simulink model "darko_control_lineaire_lqi"  (R2020b)
settings: Solver=VariableStepAuto  StartTime=0.0  StopTime=30  RelTol=1e-3
values from neighbouring files (symbols this model uses):
  drone = generateDarko()    [main_linearisation_rot.m]
  initial_state = [p_initial; v_initial; q_initial; omega_initial]    [main_linearisation_rot.m]
  K_complet_i = [Ki(:,1:6), zeros(4,1), Ki(:,7:15)]    [main_linearisation_rot.m]
  S_complet_i = [Si(1:6,1:6), zeros(6,1), Si(1:6,7:15); zeros(1,16); Si(7:15,1:6), zeros(9,1), Si(7:15,7:15)]    [main_linearisation_rot.m]
  u_eq = drone.G*drone.MASS/(2*drone.Fb(1,1)) * [1;1;0;0]    [main_linearisation_rot.m]
  x_eq = [[0; 0; 0]; [0; 0; 0]; [1/sqrt(2); 0; -1/sqrt(2);0]; [0; 0; 0]]    [main_linearisation_rot.m]
libraries: simulink_extras x5, aerolibanim x1, sharedtransform x1
settings Model: Creator=florian  LastModifiedBy=florian

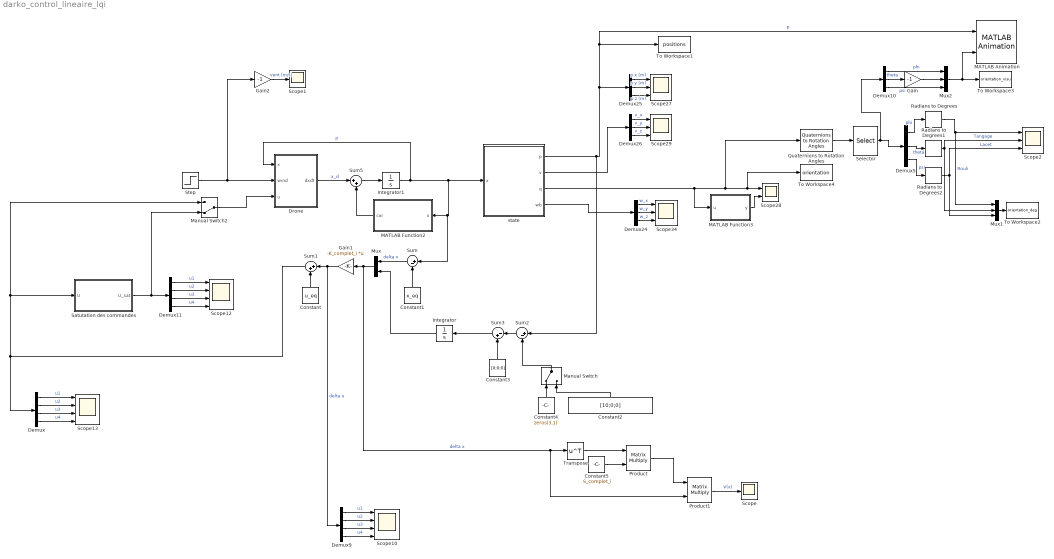
== system darko_control_lineaire_lqi ==
  Constant : Constant  Value=u_eq
  Constant1 : Constant  Value=x_eq
  Constant2 : Constant  Value=[10;0;0]
  Constant3 : Constant  Value=[0;0;0]
  Constant4 : Constant  Value=zeros(3,1)
  Constant5 : Constant  Value=S_complet_i
  Demux : Demux
  Demux{5,10,24..26} (5 alike) : Demux  Outputs=3
  Demux11 : Demux
  Demux9 : Demux
  Drone : MATLAB Function  TreatAsAtomicUnit=on
  Gain : Gain  Gain=-1
  Gain1 : Gain  Gain=-K_complet_i  Multiplication=Matrix(K*u) (u vector)
  Gain2 : Gain  Gain=-1
  Integrator : Integrator  InitialCondition=[0;0;0]
  Integrator1 : Integrator  InitialCondition=initial_state
  MATLAB Animation : aerolibanim/MATLAB Animation  Tag=Matlab Animation 6 DOF  Vehicles=1  Geometries='astredwedge.mat'  BoundingBoxCoordinates=[-50,50,-50,50,-50,50]  CameraOffset=[0,-50,0]  CameraViewAngle=10  SampleTime=0.08  FigurePosition=[635,-23,492,413]
      settings: SourceProductBaseCode=AE
  MATLAB Function2 : MATLAB Function  TreatAsAtomicUnit=on
  MATLAB Function3 : MATLAB Function  TreatAsAtomicUnit=on
  Manual Switch : ManualSwitch
  Manual Switch2 : ManualSwitch  CurrentSetting=0
  Mux : Mux  Inputs=2
  Mux1 : Mux  Inputs=3
  Mux2 : Mux  Inputs=3
  Product : Product  Multiplication=Matrix(*)
  Product1 : Product  Multiplication=Matrix(*)
  Quaternions to Rotation Angles : sharedtransform/Quaternions to Rotation Angles  rotationOrder=ZXY  aMode=aMode
      settings: SourceProductBaseCode=AE,PW,MT,UV,VE,VP
  Radians to Degrees : simulink_extras/Transformations/Radians to Degrees
  Radians to Degrees1 : simulink_extras/Transformations/Radians to Degrees
  Radians to Degrees2 : simulink_extras/Transformations/Radians to Degrees
  Satutation des commandes : Subsystem
  Scope : Scope
  Scope1 : Scope
  Scope10 : Scope  NumInputPorts=4
  Scope12 : Scope  NumInputPorts=4
  Scope13 : Scope  NumInputPorts=4
  Scope{2,27,29,34} (4 alike) : Scope  NumInputPorts=3
  Scope28 : Scope  NumInputPorts=2
  Selector : Selector  InputPortWidth=3  IndexOptions=Index vector (dialog)  Indices=[2 3 1]  OutputSizes=1
  Step : Step  Time=10  Before=[0;0;0]  After=[-5;0;0]  SampleTime=0
  Sum : Sum  Inputs=|+-
  Sum1 : Sum  Inputs=|++
  Sum2 : Sum  Inputs=|+-
  Sum3 : Sum  Inputs=|-+
  Sum5 : Sum  Inputs=|++
  To Workspace1 : ToWorkspace  VariableName=positions  SampleTime=-1
  To Workspace2 : ToWorkspace  VariableName=orientation_deg  SampleTime=-1
  To Workspace3 : ToWorkspace  VariableName=orientation_visu  SampleTime=-1
  To Workspace4 : ToWorkspace  VariableName=orientation  SampleTime=-1
  Transpose : Math  Operator=transpose  SaturateOnIntegerOverflow=on
  state : MATLAB Function  TreatAsAtomicUnit=on
  wires:
  Sum5/1 -> Integrator1/1
  MATLAB Function2/1(cor) -> Sum5/2
  Drone/1(dxdt) -> Sum5/1  "x_d"
  Integrator1/1 -> Drone/1(x), state/1(x), Sum/1, MATLAB Function2/1(x)  "p"
  Demux25/3 -> Scope27/3  "p z (m)"
  Demux26/2 -> Scope29/2  "v_y"
  Demux24/1 -> Scope34/1  "w_x"
  MATLAB Function3/1(y) -> Scope28/2
  Demux25/1 -> Scope27/1  "p x (m)"
  state/4(wb) -> Demux24/1
  Demux24/2 -> Scope34/2  "w_y"
  Demux24/3 -> Scope34/3  "w_z"
  state/2(v) -> Demux26/1
  Demux25/2 -> Scope27/2  "p y (m)"
  Demux26/3 -> Scope29/3  "v_z"
  Demux26/1 -> Scope29/1  "v_x"
  Constant/1 -> Sum1/2
  Constant1/1 -> Sum/2
  Demux9/3 -> Scope10/3  "u3"
  Demux9/4 -> Scope10/4  "u4"
  Demux9/1 -> Scope10/1  "u1"
  Demux9/2 -> Scope10/2  "u2"
  Step/1 -> Gain2/1, Drone/2(wind)
  Sum3/1 -> Integrator/1
  Constant3/1 -> Sum3/2
  Integrator/1 -> Mux/2
  Sum/1 -> Mux/1  "delta x"
  Demux5/2 -> Radians to Degrees1/1  "theta"
  Quaternions to Rotation Angles/1 -> Selector/1
  Demux5/1 -> Radians to Degrees/1  "phi"
  Demux5/3 -> Radians to Degrees2/1  "psi"
  Constant2/1 -> Manual Switch/2
  Constant4/1 -> Manual Switch/1
  Manual Switch/1 -> Sum2/2
  Sum2/1 -> Sum3/1
  Demux/3 -> Scope13/3  "u3"
  Demux11/1 -> Scope12/1  "u1"
  Demux11/2 -> Scope12/2  "u2"
  Sum1/1 -> Satutation des commandes/1(U), Manual Switch2/1, Demux/1
  Demux11/3 -> Scope12/3  "u3"
  Demux/2 -> Scope13/2  "u2"
  Manual Switch2/1 -> Drone/3(u)
  Demux/1 -> Scope13/1  "u1"
  Demux/4 -> Scope13/4  "u4"
  Demux11/4 -> Scope12/4  "u4"
  Product1/1 -> Scope/1  "V(x)"
  Gain1/1 -> Demux9/1, Sum1/1  "delta u"
  Product/1 -> Product1/1
  Transpose/1 -> Product/1
  Constant5/1 -> Product/2
  Mux/1 -> Product1/2, Transpose/1, Gain1/1  "delta x"
  Mux1/1 -> To Workspace2/1
  state/3(q) -> Scope28/1, To Workspace4/1, Quaternions to Rotation Angles/1, MATLAB Function3/1(u)
  Satutation des commandes/1(U_sat) -> Manual Switch2/2, Demux11/1
  Demux10/2 -> Gain/1  "theta"
  Selector/1 -> Demux10/1, Demux5/1
  Gain/1 -> Mux2/2
  Demux10/1 -> Mux2/1  "phi"
  Demux10/3 -> Mux2/3  "psi"
  state/1(p) -> Sum2/1, Demux25/1, MATLAB Animation/1, To Workspace1/1  "p"
  Mux2/1 -> To Workspace3/1, MATLAB Animation/2
  Gain2/1 -> Scope1/1  "vent (m/s)"
  Radians to Degrees1/1 -> Scope2/2, Mux1/2  "Tangage"
  Radians to Degrees/1 -> Scope2/1, Mux1/1  "Rouli"
  Radians to Degrees2/1 -> Scope2/3, Mux1/3  "Lacet"

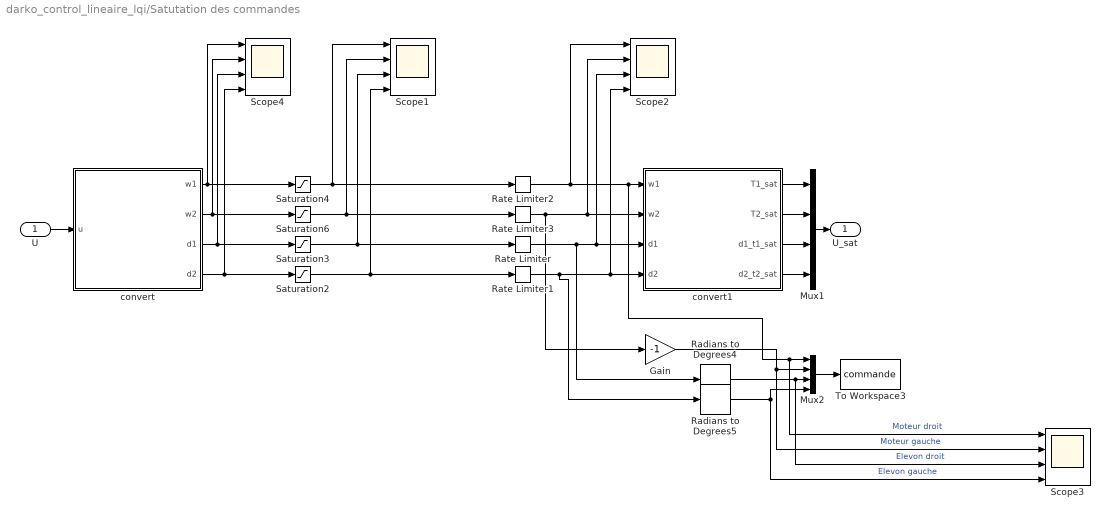
== system darko_control_lineaire_lqi/Satutation des commandes ==
  U : Inport
  Gain : Gain  Gain=-1
  Mux1 : Mux
  Mux2 : Mux
  Radians to Degrees4 : simulink_extras/Transformations/Radians to Degrees
  Radians to Degrees5 : simulink_extras/Transformations/Radians to Degrees
  Rate Limiter : RateLimiter  RisingSlewLimit=drone.ELEVON_RATE_CHANGE  FallingSlewLimit=-drone.ELEVON_RATE_CHANGE  SampleTimeMode=inherited
  Rate Limiter1 : RateLimiter  RisingSlewLimit=drone.ELEVON_RATE_CHANGE  FallingSlewLimit=-drone.ELEVON_RATE_CHANGE  SampleTimeMode=inherited
  Rate Limiter2 : RateLimiter  RisingSlewLimit=drone.MOTOR_RATE_CHANGE  FallingSlewLimit=-drone.MOTOR_RATE_CHANGE  SampleTimeMode=inherited
  Rate Limiter3 : RateLimiter  RisingSlewLimit=drone.MOTOR_RATE_CHANGE  FallingSlewLimit=-drone.MOTOR_RATE_CHANGE  SampleTimeMode=inherited
  Saturation2 : Saturate  UpperLimit=30*(pi/180)  LowerLimit=-30*(pi/180)
  Saturation3 : Saturate  UpperLimit=30*(pi/180)  LowerLimit=-30*(pi/180)
  Saturation4 : Saturate  UpperLimit=1000  LowerLimit=200
  Saturation6 : Saturate  UpperLimit=1000  LowerLimit=200
  Scope{1..4} (4 alike) : Scope  NumInputPorts=4
  To Workspace3 : ToWorkspace  VariableName=commande  SampleTime=-1
  convert : MATLAB Function  TreatAsAtomicUnit=on
  convert1 : MATLAB Function  TreatAsAtomicUnit=on
  U_sat : Outport
  wires:
  convert/1(w1) -> Saturation4/1, Scope4/1
  Saturation3/1 -> Rate Limiter/1, Scope1/3
  convert/2(w2) -> Scope4/2, Saturation6/1
  convert/3(d1) -> Scope4/3, Saturation3/1
  convert/4(d2) -> Saturation2/1, Scope4/4
  convert1/1(T1_sat) -> Mux1/1
  convert1/4(d2_t2_sat) -> Mux1/4
  Mux1/1 -> U_sat/1
  convert1/2(T2_sat) -> Mux1/2
  convert1/3(d1_t1_sat) -> Mux1/3
  Saturation2/1 -> Rate Limiter1/1, Scope1/4
  Saturation6/1 -> Rate Limiter3/1, Scope1/2
  Saturation4/1 -> Rate Limiter2/1, Scope1/1
  U/1 -> convert/1(u)
  Radians to Degrees5/1 -> Mux2/4, Scope3/4  "Elevon gauche"
  Rate Limiter3/1 -> Gain/1, convert1/2(w2), Scope2/2
  Rate Limiter1/1 -> Radians to Degrees5/1, Scope2/4, convert1/4(d2)
  Rate Limiter/1 -> Radians to Degrees4/1, Scope2/3, convert1/3(d1)
  Gain/1 -> Scope3/2, Mux2/2  "Moteur gauche"
  Mux2/1 -> To Workspace3/1
  Radians to Degrees4/1 -> Scope3/3, Mux2/3  "Elevon droit"
  Rate Limiter2/1 -> Scope2/1, Scope3/1, Mux2/1, convert1/1(w1)  "Moteur droit"

== matlab function darko_control_lineaire_lqi/Drone ==
  data: x input; wind input; u input; dxdt output; drone parameter
function dxdt  = drone(x,wind, u, drone)

%% physical constants
% gravity
g = drone.G;
% vehicle mass
m = drone.MASS;
% vehicle inertia matrix
J = drone.INERTIA; % [3x3 real symmetric] in body axis

%% state demultiplexing
% p = x(1:3);
v = x(4:6);
q  = x(7:10);
wb = x(11:13);

Rq = q2dcm(q);

[Fp, Mp] = external_force_moment(x, u, wind, drone);

% position
dpdt = v;

% kinematics
dvdt =  -[0;0;g] + (1/m)*Rq*drone.Fb*u + (1/m)*Rq*Fp; 

%% quaternion derivative
eta = q(1);
eps = q(2:4);

dqdt = (1/2)*[-eps'; eta*eye(3) + skew_sym(eps)]*wb;

%% angular velocity derivative
% kinematics
dwdt = -J\cross(wb, J*wb) + J\(drone.Mb*u) + J\Mp;


%% derivative multiplexing
dxdt = [dpdt; dvdt; dqdt; dwdt] ;

== matlab function darko_control_lineaire_lqi/Satutation des commandes/convert ==
  data: u input; w1 output; drone parameter; w2 output; d1 output; d2 output
function [w1, w2, d1, d2] = convert(u, drone)
%#codegen
kf = drone.PROP_KP;

T1 = max(u(1),0);
T2 = max(u(2),0);
d1_T1 = u(3);
d2_T2 = u(4);

w1 = sqrt(T1/kf);
w2 = sqrt(T2/kf);
d1 = d1_T1/T1;
d2 = d2_T2/T2;

== matlab function darko_control_lineaire_lqi/Satutation des commandes/convert1 ==
  data: w1 input; w2 input; d1 input; d2 input; T1_sat output; T2_sat output; drone parameter; d1_t1_sat output; d2_t2_sat output
function [T1_sat, T2_sat, d1_t1_sat, d2_t2_sat] = convert2(w1, w2, d1, d2, drone)
%#codegen
kf = drone.PROP_KP;

T1_sat = kf*w1^2;
d1_t1_sat = d1*T1_sat;
T2_sat = kf*w2^2;
d2_t2_sat = d2*T2_sat;

== matlab function darko_control_lineaire_lqi/MATLAB Function2 ==
  data: x input; cor output
function cor  = fcn(x)
%#codegen
q  = x(7:10);
n = norm(q);
mismatch = 1-n;
cor = [0;0;0; 0;0;0; mismatch*q; 0;0;0];

== matlab function darko_control_lineaire_lqi/MATLAB Function3 ==
  data: u input; y output
function y = fcn(u)
%#codegen

y = norm(u);

== matlab function darko_control_lineaire_lqi/state ==
  data: x input; p output; v output; q output; wb output
function [p, v, q, wb] = demux(x)
%#codegen

p = x(1:3);
v = x(4:6);
q  = x(7:10);
wb = x(11:13);
